simulink model "Suma"  (R2013b)
settings: Solver=ode3  StartTime=0.0  StopTime=5.0  FixedStep=0.001  RelTol=1e-3
settings Model: Creator=LAB1-8  LastModifiedBy=LAB1-8

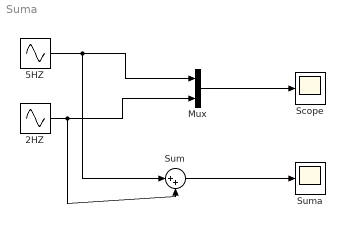
== system Suma ==
  2HZ : Sin  Amplitude=10  Frequency=2*2*pi  Phase=pi/2  SampleTime=0
  5HZ : Sin  Amplitude=10  Frequency=5*2*pi  Phase=pi/2  SampleTime=0
  Mux : Mux  Inputs=2
  Scope : Scope
      settings: ShowLegends=on  MaxDataPoints=5000000
  Sum : Sum  Inputs=|++
  Suma : Scope
      settings: ShowLegends=on  MaxDataPoints=5000000
  wires:
  5HZ/1 -> Sum/1, Mux/1
  2HZ/1 -> Sum/2, Mux/2
  Mux/1 -> Scope/1
  Sum/1 -> Suma/1
